simulink model "satellite_sim"  (R2019b)
settings: Solver=VariableStepAuto  StartTime=0.0  StopTime=10.0  RelTol=1e-3
InitFcn:
  | restoredefaultpath
  | clear all
  | addpath ./..
  | satelliteParam
undefined symbols (not defined in the file): P, satellite_animation
settings Model: Creator=JoHn  LastModifiedBy=JoHn

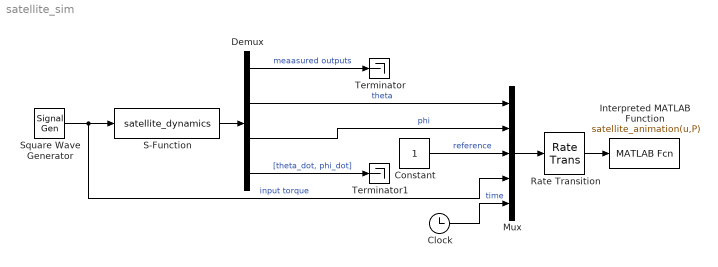
== system satellite_sim ==
  Clock : Clock
  Constant : Constant
  Demux : Demux  Outputs=[2,1,1,2]
  Interpreted MATLAB Function : MATLABFcn  MATLABFcn=satellite_animation(u,P)  OutputDimensions=0
  Mux : Mux  Inputs=5
  Rate Transition : RateTransition  OutPortSampleTime=P.t_plot
  S-Function : S-Function  FunctionName=satellite_dynamics  Parameters=P  SFunctionDeploymentMode=off  EnableBusSupport=off
  Square Wave Generator : SignalGenerator  WaveForm=square  Units=rad/sec
  Terminator : Terminator
  Terminator1 : Terminator
  wires:
  Square Wave Generator/1 -> Mux/4, S-Function/1  "input torque"
  S-Function/1 -> Demux/1
  Demux/1 -> Terminator/1  "meaasured outputs"
  Demux/4 -> Terminator1/1  "[theta_dot, phi_dot]"
  Demux/2 -> Mux/1  "theta"
  Demux/3 -> Mux/2  "phi"
  Constant/1 -> Mux/3  "reference"
  Clock/1 -> Mux/5  "time"
  Mux/1 -> Rate Transition/1
  Rate Transition/1 -> Interpreted MATLAB Function/1
